simulink model "RCAMSimulation"  (R2024a)
settings: Solver=VariableStepAuto  StartTime=0.0  StopTime=TF  RelTol=1e-3
values from neighbouring files (symbols this model uses):
  umax = deg2rad(umax)    [Initialize.m]
  umin = deg2rad(umin)    [Initialize.m]
  x0 = [85 ... (first row only)    [Initialize.m]
undefined symbols (not defined in the file or in its folder): RCAM_model
settings Model: Creator=Kartik Parameshwaran  LastModifiedBy=Kartik Parameshwaran

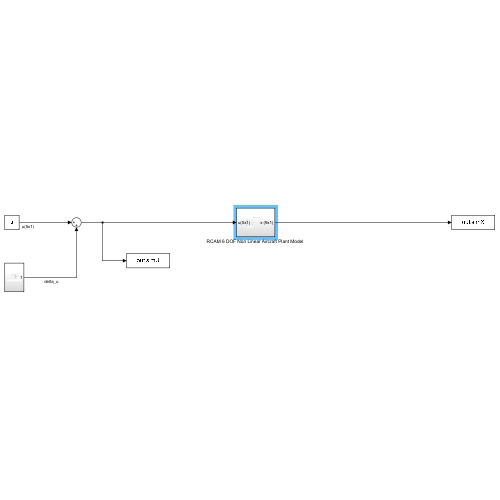
[thumbnail: Simulink's stored preview of the top-level diagram]
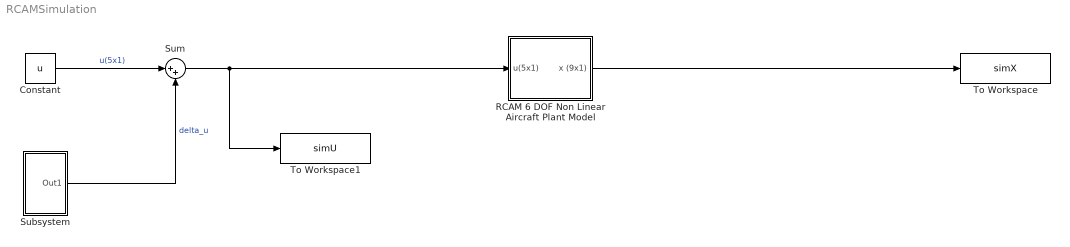
== system RCAMSimulation ==
  Constant : Constant  Value=u
  "RCAM 6 DOF Non Linear Aircraft Plant Model " : Subsystem
  Subsystem : Subsystem
  Sum : Sum  Inputs=|++
  To Workspace : ToWorkspace  VariableName=simX  SaveFormat=Timeseries  SampleTime=-1
  To Workspace1 : ToWorkspace  VariableName=simU  SaveFormat=Timeseries  SampleTime=-1
  wires:
  "RCAM 6 DOF Non Linear Aircraft Plant Model "/1(x (9x1)) -> To Workspace/1
  Constant/1 -> Sum/1  "u(5x1)"
  Subsystem/1(Out1) -> Sum/2  "delta_u"
  Sum/1 -> To Workspace1/1, "RCAM 6 DOF Non Linear Aircraft Plant Model "/1(u(5x1))

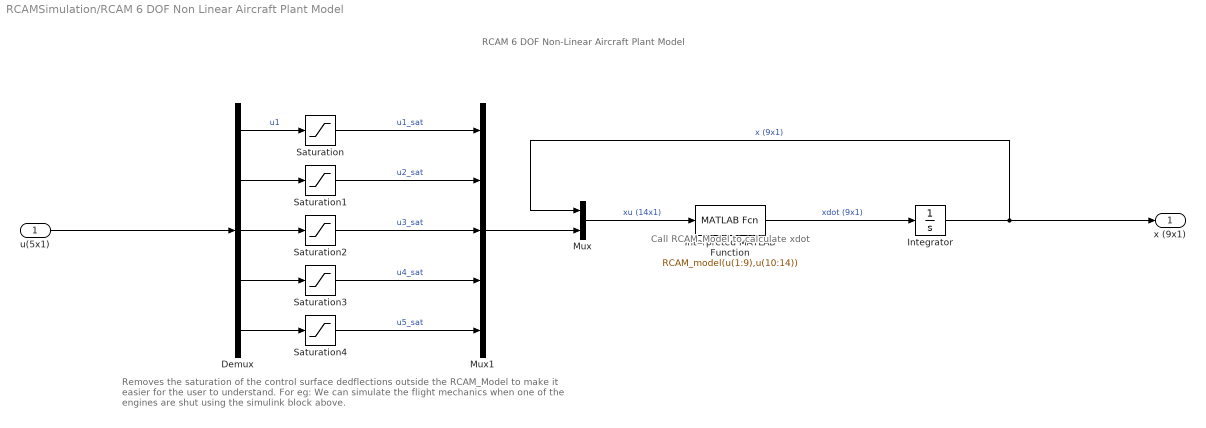
== system RCAMSimulation/RCAM 6 DOF Non Linear Aircraft Plant Model  ==
  note: RCAM 6 DOF Non-Linear Aircraft Plant Model
  note: Removes the saturation of the control surface dedflections outside the RCAM_Model to make it easier for the user to understand.
      |
      | For eg: We can simulate the flight mechanics when one of the engines are shut using the simulink block above.
  note: Call RCAM_Model to calculate xdot
  u(5x1) : Inport
  Demux : Demux  Outputs=5
  Integrator : Integrator  InitialCondition=x0
  Interpreted MATLAB Function : MATLABFcn  MATLABFcn=RCAM_model(u(1:9),u(10:14))
  Mux : Mux  Inputs=2
  Mux1 : Mux  Inputs=5
  Saturation : Saturate  UpperLimit=umax(1)  LowerLimit=umin(1)
  Saturation1 : Saturate  UpperLimit=umax(2)  LowerLimit=umin(2)
  Saturation2 : Saturate  UpperLimit=umax(3)  LowerLimit=umin(3)
  Saturation3 : Saturate  UpperLimit=umax(4)  LowerLimit=umin(4)
  Saturation4 : Saturate  UpperLimit=umax(5)  LowerLimit=umin(5)
  x (9x1) : Outport
  wires:
  u(5x1)/1 -> Demux/1
  Interpreted MATLAB Function/1 -> Integrator/1  "xdot (9x1)"
  Mux/1 -> Interpreted MATLAB Function/1  "xu (14x1)"
  Integrator/1 -> x (9x1)/1, Mux/1  "x (9x1)"
  Demux/1 -> Saturation/1  "u1"
  Saturation/1 -> Mux1/1  "u1_sat"
  Demux/2 -> Saturation1/1
  Demux/3 -> Saturation2/1
  Demux/4 -> Saturation3/1
  Demux/5 -> Saturation4/1
  Saturation1/1 -> Mux1/2  "u2_sat"
  Saturation2/1 -> Mux1/3  "u3_sat"
  Saturation3/1 -> Mux1/4  "u4_sat"
  Saturation4/1 -> Mux1/5  "u5_sat"
  Mux1/1 -> Mux/2

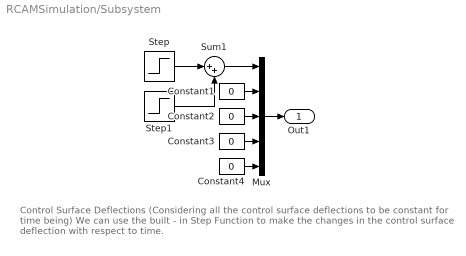
== system RCAMSimulation/Subsystem ==
  note: Control Surface Deflections (Considering all the control surface deflections to be constant for time being)
      | We can use the built - in Step Function to make the changes in the control surface deflection with respect to time.
  Constant{1..4} (4 alike) : Constant  Value=0
  Mux : Mux  Inputs=5
  Step : Step  Time=30  After=0  SampleTime=0
  Step1 : Step  Time=30+2  After=0  SampleTime=0
  Sum1 : Sum  Inputs=|++
  Out1 : Outport
  wires:
  Step1/1 -> Sum1/2
  Sum1/1 -> Mux/1
  Constant4/1 -> Mux/5
  Step/1 -> Sum1/1
  Mux/1 -> Out1/1
  Constant2/1 -> Mux/3
  Constant1/1 -> Mux/2
  Constant3/1 -> Mux/4
